simulink model "AVIC_model"  (R2015b)
settings: Solver=ode45  StartTime=0.0  StopTime=simtime  RelTol=1e-3
values from neighbouring files (symbols this model uses):
  A = 1    [simulation.m]
  a1 = 1    [simulation.m]
  a2 = 3    [simulation.m]
  a3 = 3    [simulation.m]
  Amp1 = Ampl/1000000    (= 134.217728)    [simulation.m]
  b1 = 1    [simulation.m]
  B2 = 8    [simulation.m]
  C = 32    [simulation.m]
  c1 = 1    [simulation.m]
  c2 = 1    [simulation.m]
  c3 = 1    [simulation.m]
  finrad = 2*pi/(N)*f0*clk    [simulation.m]
  FSC = 2^27    (= 134217728)    [simulation.m]
  SAT = 127    [simulation.m]
  Ts = 1/clk    (= 1.62760416667e-07)    [simulation.m]
libraries: simulink x298
(part 5 of 5)

== system AVIC_model/2値3次 NSDEM/NSDEM_3rd/Sort16/XSW23 ==
  IP : Inport
  IM : Inport  Port=2
  SP : Inport  Port=3
  SM : Inport  Port=4
  Relational Operator : RelationalOperator  Operator=<  OutDataTypeStr=boolean
  Switch{,1..3} (4 alike) : Switch  Criteria=u2 > Threshold
  OA : Outport
  OB : Outport  Port=2
  QA : Outport  Port=3
  QB : Outport  Port=4
  wires:
  IP/1 -> Relational Operator/1, Switch/1, Switch1/3
  IM/1 -> Relational Operator/2, Switch1/1, Switch/3
  Relational Operator/1 -> Switch/2, Switch1/2, Switch2/2, Switch3/2
  Switch/1 -> OA/1
  Switch1/1 -> OB/1
  SP/1 -> Switch3/3, Switch2/1
  SM/1 -> Switch3/1, Switch2/3
  Switch2/1 -> QA/1
  Switch3/1 -> QB/1

== system AVIC_model/2値3次 NSDEM/NSDEM_3rd/Sort16/XSW24 ==
  IP : Inport
  IM : Inport  Port=2
  SP : Inport  Port=3
  SM : Inport  Port=4
  Relational Operator : RelationalOperator  Operator=<  OutDataTypeStr=boolean
  Switch{,1..3} (4 alike) : Switch  Criteria=u2 > Threshold
  OA : Outport
  OB : Outport  Port=2
  QA : Outport  Port=3
  QB : Outport  Port=4
  wires:
  Switch3/1 -> QB/1
  Switch2/1 -> QA/1
  SM/1 -> Switch2/3, Switch3/1
  SP/1 -> Switch2/1, Switch3/3
  Switch1/1 -> OB/1
  Switch/1 -> OA/1
  Relational Operator/1 -> Switch3/2, Switch2/2, Switch1/2, Switch/2
  IM/1 -> Switch/3, Switch1/1, Relational Operator/2
  IP/1 -> Switch1/3, Switch/1, Relational Operator/1

== system AVIC_model/2値3次 NSDEM/NSDEM_3rd/Sort16/XSW25 ==
  IM : Inport
  IP : Inport  Port=2
  SM : Inport  Port=3
  SP : Inport  Port=4
  Relational Operator : RelationalOperator  Operator=<  OutDataTypeStr=boolean
  Switch{,1..3} (4 alike) : Switch  Criteria=u2 > Threshold
  OB : Outport
  OA : Outport  Port=2
  QB : Outport  Port=3
  QA : Outport  Port=4
  wires:
  IP/1 -> Relational Operator/1, Switch/1, Switch1/3
  IM/1 -> Relational Operator/2, Switch1/1, Switch/3
  Relational Operator/1 -> Switch/2, Switch1/2, Switch2/2, Switch3/2
  Switch/1 -> OA/1
  Switch1/1 -> OB/1
  SP/1 -> Switch3/3, Switch2/1
  SM/1 -> Switch3/1, Switch2/3
  Switch2/1 -> QA/1
  Switch3/1 -> QB/1

== system AVIC_model/2値3次 NSDEM/NSDEM_3rd/Sort16/XSW26 ==
  IM : Inport
  IP : Inport  Port=2
  SM : Inport  Port=3
  SP : Inport  Port=4
  Relational Operator : RelationalOperator  Operator=<  OutDataTypeStr=boolean
  Switch{,1..3} (4 alike) : Switch  Criteria=u2 > Threshold
  OB : Outport
  OA : Outport  Port=2
  QB : Outport  Port=3
  QA : Outport  Port=4
  wires:
  IP/1 -> Relational Operator/1, Switch/1, Switch1/3
  IM/1 -> Relational Operator/2, Switch1/1, Switch/3
  Relational Operator/1 -> Switch/2, Switch1/2, Switch2/2, Switch3/2
  Switch/1 -> OA/1
  Switch1/1 -> OB/1
  SP/1 -> Switch3/3, Switch2/1
  SM/1 -> Switch3/1, Switch2/3
  Switch2/1 -> QA/1
  Switch3/1 -> QB/1

== system AVIC_model/2値3次 NSDEM/NSDEM_3rd/Sort16/XSW27 ==
  IM : Inport
  IP : Inport  Port=2
  SM : Inport  Port=3
  SP : Inport  Port=4
  Relational Operator : RelationalOperator  Operator=<  OutDataTypeStr=boolean
  Switch{,1..3} (4 alike) : Switch  Criteria=u2 > Threshold
  OB : Outport
  OA : Outport  Port=2
  QB : Outport  Port=3
  QA : Outport  Port=4
  wires:
  Switch3/1 -> QB/1
  Switch2/1 -> QA/1
  SM/1 -> Switch2/3, Switch3/1
  SP/1 -> Switch2/1, Switch3/3
  Switch1/1 -> OB/1
  Switch/1 -> OA/1
  Relational Operator/1 -> Switch3/2, Switch2/2, Switch1/2, Switch/2
  IM/1 -> Switch/3, Switch1/1, Relational Operator/2
  IP/1 -> Switch1/3, Switch/1, Relational Operator/1

== system AVIC_model/2値3次 NSDEM/NSDEM_3rd/Sort16/XSW28 ==
  IM : Inport
  IP : Inport  Port=2
  SM : Inport  Port=3
  SP : Inport  Port=4
  Relational Operator : RelationalOperator  Operator=<  OutDataTypeStr=boolean
  Switch{,1..3} (4 alike) : Switch  Criteria=u2 > Threshold
  OB : Outport
  OA : Outport  Port=2
  QB : Outport  Port=3
  QA : Outport  Port=4
  wires:
  Switch3/1 -> QB/1
  Switch2/1 -> QA/1
  SM/1 -> Switch2/3, Switch3/1
  SP/1 -> Switch2/1, Switch3/3
  Switch1/1 -> OB/1
  Switch/1 -> OA/1
  Relational Operator/1 -> Switch3/2, Switch2/2, Switch1/2, Switch/2
  IM/1 -> Switch/3, Switch1/1, Relational Operator/2
  IP/1 -> Switch1/3, Switch/1, Relational Operator/1

== system AVIC_model/2値3次 NSDEM/NSDEM_3rd/Sort16/XSW29 ==
  IM : Inport
  IP : Inport  Port=2
  SM : Inport  Port=3
  SP : Inport  Port=4
  Relational Operator : RelationalOperator  Operator=<  OutDataTypeStr=boolean
  Switch{,1..3} (4 alike) : Switch  Criteria=u2 > Threshold
  OB : Outport
  OA : Outport  Port=2
  QB : Outport  Port=3
  QA : Outport  Port=4
  wires:
  Switch3/1 -> QB/1
  Switch2/1 -> QA/1
  SM/1 -> Switch2/3, Switch3/1
  SP/1 -> Switch2/1, Switch3/3
  Switch1/1 -> OB/1
  Switch/1 -> OA/1
  Relational Operator/1 -> Switch3/2, Switch2/2, Switch1/2, Switch/2
  IM/1 -> Switch/3, Switch1/1, Relational Operator/2
  IP/1 -> Switch1/3, Switch/1, Relational Operator/1

== system AVIC_model/2値3次 NSDEM/NSDEM_3rd/Sort16/XSW3 ==
  IM : Inport
  IP : Inport  Port=2
  SM : Inport  Port=3
  SP : Inport  Port=4
  Relational Operator : RelationalOperator  Operator=<  OutDataTypeStr=boolean
  Switch{,1..3} (4 alike) : Switch  Criteria=u2 > Threshold
  OB : Outport
  OA : Outport  Port=2
  QB : Outport  Port=3
  QA : Outport  Port=4
  wires:
  Switch3/1 -> QB/1
  Switch2/1 -> QA/1
  SM/1 -> Switch2/3, Switch3/1
  SP/1 -> Switch2/1, Switch3/3
  Switch1/1 -> OB/1
  Switch/1 -> OA/1
  Relational Operator/1 -> Switch3/2, Switch2/2, Switch1/2, Switch/2
  IM/1 -> Switch/3, Switch1/1, Relational Operator/2
  IP/1 -> Switch1/3, Switch/1, Relational Operator/1

== system AVIC_model/2値3次 NSDEM/NSDEM_3rd/Sort16/XSW30 ==
  IM : Inport
  IP : Inport  Port=2
  SM : Inport  Port=3
  SP : Inport  Port=4
  Relational Operator : RelationalOperator  Operator=<  OutDataTypeStr=boolean
  Switch{,1..3} (4 alike) : Switch  Criteria=u2 > Threshold
  OB : Outport
  OA : Outport  Port=2
  QB : Outport  Port=3
  QA : Outport  Port=4
  wires:
  Switch3/1 -> QB/1
  Switch2/1 -> QA/1
  SM/1 -> Switch2/3, Switch3/1
  SP/1 -> Switch2/1, Switch3/3
  Switch1/1 -> OB/1
  Switch/1 -> OA/1
  Relational Operator/1 -> Switch3/2, Switch2/2, Switch1/2, Switch/2
  IM/1 -> Switch/3, Switch1/1, Relational Operator/2
  IP/1 -> Switch1/3, Switch/1, Relational Operator/1

== system AVIC_model/2値3次 NSDEM/NSDEM_3rd/Sort16/XSW31 ==
  IM : Inport
  IP : Inport  Port=2
  SM : Inport  Port=3
  SP : Inport  Port=4
  Relational Operator : RelationalOperator  Operator=<  OutDataTypeStr=boolean
  Switch{,1..3} (4 alike) : Switch  Criteria=u2 > Threshold
  OB : Outport
  OA : Outport  Port=2
  QB : Outport  Port=3
  QA : Outport  Port=4
  wires:
  Switch3/1 -> QB/1
  Switch2/1 -> QA/1
  SM/1 -> Switch2/3, Switch3/1
  SP/1 -> Switch2/1, Switch3/3
  Switch1/1 -> OB/1
  Switch/1 -> OA/1
  Relational Operator/1 -> Switch3/2, Switch2/2, Switch1/2, Switch/2
  IM/1 -> Switch/3, Switch1/1, Relational Operator/2
  IP/1 -> Switch1/3, Switch/1, Relational Operator/1

== system AVIC_model/2値3次 NSDEM/NSDEM_3rd/Sort16/XSW32 ==
  IM : Inport
  IP : Inport  Port=2
  SM : Inport  Port=3
  SP : Inport  Port=4
  Relational Operator : RelationalOperator  Operator=<  OutDataTypeStr=boolean
  Switch{,1..3} (4 alike) : Switch  Criteria=u2 > Threshold
  OB : Outport
  OA : Outport  Port=2
  QB : Outport  Port=3
  QA : Outport  Port=4
  wires:
  Switch3/1 -> QB/1
  Switch2/1 -> QA/1
  SM/1 -> Switch2/3, Switch3/1
  SP/1 -> Switch2/1, Switch3/3
  Switch1/1 -> OB/1
  Switch/1 -> OA/1
  Relational Operator/1 -> Switch3/2, Switch2/2, Switch1/2, Switch/2
  IM/1 -> Switch/3, Switch1/1, Relational Operator/2
  IP/1 -> Switch1/3, Switch/1, Relational Operator/1

== system AVIC_model/2値3次 NSDEM/NSDEM_3rd/Sort16/XSW33 ==
  IM : Inport
  IP : Inport  Port=2
  SM : Inport  Port=3
  SP : Inport  Port=4
  Relational Operator : RelationalOperator  Operator=<  OutDataTypeStr=boolean
  Switch{,1..3} (4 alike) : Switch  Criteria=u2 > Threshold
  OB : Outport
  OA : Outport  Port=2
  QB : Outport  Port=3
  QA : Outport  Port=4
  wires:
  Switch3/1 -> QB/1
  Switch2/1 -> QA/1
  SM/1 -> Switch2/3, Switch3/1
  SP/1 -> Switch2/1, Switch3/3
  Switch1/1 -> OB/1
  Switch/1 -> OA/1
  Relational Operator/1 -> Switch3/2, Switch2/2, Switch1/2, Switch/2
  IM/1 -> Switch/3, Switch1/1, Relational Operator/2
  IP/1 -> Switch1/3, Switch/1, Relational Operator/1

== system AVIC_model/2値3次 NSDEM/NSDEM_3rd/Sort16/XSW34 ==
  IM : Inport
  IP : Inport  Port=2
  SM : Inport  Port=3
  SP : Inport  Port=4
  Relational Operator : RelationalOperator  Operator=<  OutDataTypeStr=boolean
  Switch{,1..3} (4 alike) : Switch  Criteria=u2 > Threshold
  OB : Outport
  OA : Outport  Port=2
  QB : Outport  Port=3
  QA : Outport  Port=4
  wires:
  Switch3/1 -> QB/1
  Switch2/1 -> QA/1
  SM/1 -> Switch2/3, Switch3/1
  SP/1 -> Switch2/1, Switch3/3
  Switch1/1 -> OB/1
  Switch/1 -> OA/1
  Relational Operator/1 -> Switch3/2, Switch2/2, Switch1/2, Switch/2
  IM/1 -> Switch/3, Switch1/1, Relational Operator/2
  IP/1 -> Switch1/3, Switch/1, Relational Operator/1

== system AVIC_model/2値3次 NSDEM/NSDEM_3rd/Sort16/XSW35 ==
  IM : Inport
  IP : Inport  Port=2
  SM : Inport  Port=3
  SP : Inport  Port=4
  Relational Operator : RelationalOperator  Operator=<  OutDataTypeStr=boolean
  Switch{,1..3} (4 alike) : Switch  Criteria=u2 > Threshold
  OB : Outport
  OA : Outport  Port=2
  QB : Outport  Port=3
  QA : Outport  Port=4
  wires:
  Switch3/1 -> QB/1
  Switch2/1 -> QA/1
  SM/1 -> Switch2/3, Switch3/1
  SP/1 -> Switch2/1, Switch3/3
  Switch1/1 -> OB/1
  Switch/1 -> OA/1
  Relational Operator/1 -> Switch3/2, Switch2/2, Switch1/2, Switch/2
  IM/1 -> Switch/3, Switch1/1, Relational Operator/2
  IP/1 -> Switch1/3, Switch/1, Relational Operator/1

== system AVIC_model/2値3次 NSDEM/NSDEM_3rd/Sort16/XSW36 ==
  IP : Inport
  IM : Inport  Port=2
  SP : Inport  Port=3
  SM : Inport  Port=4
  Relational Operator : RelationalOperator  Operator=<  OutDataTypeStr=boolean
  Switch{,1..3} (4 alike) : Switch  Criteria=u2 > Threshold
  OA : Outport
  OB : Outport  Port=2
  QA : Outport  Port=3
  QB : Outport  Port=4
  wires:
  IP/1 -> Relational Operator/1, Switch/1, Switch1/3
  IM/1 -> Relational Operator/2, Switch1/1, Switch/3
  Relational Operator/1 -> Switch/2, Switch1/2, Switch2/2, Switch3/2
  Switch/1 -> OA/1
  Switch1/1 -> OB/1
  SP/1 -> Switch3/3, Switch2/1
  SM/1 -> Switch3/1, Switch2/3
  Switch2/1 -> QA/1
  Switch3/1 -> QB/1

== system AVIC_model/2値3次 NSDEM/NSDEM_3rd/Sort16/XSW37 ==
  IM : Inport
  IP : Inport  Port=2
  SM : Inport  Port=3
  SP : Inport  Port=4
  Relational Operator : RelationalOperator  Operator=<  OutDataTypeStr=boolean
  Switch{,1..3} (4 alike) : Switch  Criteria=u2 > Threshold
  OB : Outport
  OA : Outport  Port=2
  QB : Outport  Port=3
  QA : Outport  Port=4
  wires:
  Switch3/1 -> QB/1
  Switch2/1 -> QA/1
  SM/1 -> Switch2/3, Switch3/1
  SP/1 -> Switch2/1, Switch3/3
  Switch1/1 -> OB/1
  Switch/1 -> OA/1
  Relational Operator/1 -> Switch3/2, Switch2/2, Switch1/2, Switch/2
  IM/1 -> Switch/3, Switch1/1, Relational Operator/2
  IP/1 -> Switch1/3, Switch/1, Relational Operator/1

== system AVIC_model/2値3次 NSDEM/NSDEM_3rd/Sort16/XSW38 ==
  IM : Inport
  IP : Inport  Port=2
  SM : Inport  Port=3
  SP : Inport  Port=4
  Relational Operator : RelationalOperator  Operator=<  OutDataTypeStr=boolean
  Switch{,1..3} (4 alike) : Switch  Criteria=u2 > Threshold
  OB : Outport
  OA : Outport  Port=2
  QB : Outport  Port=3
  QA : Outport  Port=4
  wires:
  Switch3/1 -> QB/1
  Switch2/1 -> QA/1
  SM/1 -> Switch2/3, Switch3/1
  SP/1 -> Switch2/1, Switch3/3
  Switch1/1 -> OB/1
  Switch/1 -> OA/1
  Relational Operator/1 -> Switch3/2, Switch2/2, Switch1/2, Switch/2
  IM/1 -> Switch/3, Switch1/1, Relational Operator/2
  IP/1 -> Switch1/3, Switch/1, Relational Operator/1

== system AVIC_model/2値3次 NSDEM/NSDEM_3rd/Sort16/XSW39 ==
  IP : Inport
  IM : Inport  Port=2
  SP : Inport  Port=3
  SM : Inport  Port=4
  Relational Operator : RelationalOperator  Operator=<  OutDataTypeStr=boolean
  Switch{,1..3} (4 alike) : Switch  Criteria=u2 > Threshold
  OA : Outport
  OB : Outport  Port=2
  QA : Outport  Port=3
  QB : Outport  Port=4
  wires:
  Switch3/1 -> QB/1
  Switch2/1 -> QA/1
  SM/1 -> Switch2/3, Switch3/1
  SP/1 -> Switch2/1, Switch3/3
  Switch1/1 -> OB/1
  Switch/1 -> OA/1
  Relational Operator/1 -> Switch3/2, Switch2/2, Switch1/2, Switch/2
  IM/1 -> Switch/3, Switch1/1, Relational Operator/2
  IP/1 -> Switch1/3, Switch/1, Relational Operator/1

== system AVIC_model/2値3次 NSDEM/NSDEM_3rd/Sort16/XSW4 ==
  IP : Inport
  IM : Inport  Port=2
  SP : Inport  Port=3
  SM : Inport  Port=4
  Relational Operator : RelationalOperator  Operator=<  OutDataTypeStr=boolean
  Switch{,1..3} (4 alike) : Switch  Criteria=u2 > Threshold
  OA : Outport
  OB : Outport  Port=2
  QA : Outport  Port=3
  QB : Outport  Port=4
  wires:
  IP/1 -> Relational Operator/1, Switch/1, Switch1/3
  IM/1 -> Relational Operator/2, Switch1/1, Switch/3
  Relational Operator/1 -> Switch/2, Switch1/2, Switch2/2, Switch3/2
  Switch/1 -> OA/1
  Switch1/1 -> OB/1
  SP/1 -> Switch3/3, Switch2/1
  SM/1 -> Switch3/1, Switch2/3
  Switch2/1 -> QA/1
  Switch3/1 -> QB/1

== system AVIC_model/2値3次 NSDEM/NSDEM_3rd/Sort16/XSW40 ==
  IP : Inport
  IM : Inport  Port=2
  SP : Inport  Port=3
  SM : Inport  Port=4
  Relational Operator : RelationalOperator  Operator=<  OutDataTypeStr=boolean
  Switch{,1..3} (4 alike) : Switch  Criteria=u2 > Threshold
  OA : Outport
  OB : Outport  Port=2
  QA : Outport  Port=3
  QB : Outport  Port=4
  wires:
  Switch3/1 -> QB/1
  Switch2/1 -> QA/1
  SM/1 -> Switch2/3, Switch3/1
  SP/1 -> Switch2/1, Switch3/3
  Switch1/1 -> OB/1
  Switch/1 -> OA/1
  Relational Operator/1 -> Switch3/2, Switch2/2, Switch1/2, Switch/2
  IM/1 -> Switch/3, Switch1/1, Relational Operator/2
  IP/1 -> Switch1/3, Switch/1, Relational Operator/1

== system AVIC_model/2値3次 NSDEM/NSDEM_3rd/Sort16/XSW41 ==
  IM : Inport
  IP : Inport  Port=2
  SM : Inport  Port=3
  SP : Inport  Port=4
  Relational Operator : RelationalOperator  Operator=<  OutDataTypeStr=boolean
  Switch{,1..3} (4 alike) : Switch  Criteria=u2 > Threshold
  OB : Outport
  OA : Outport  Port=2
  QB : Outport  Port=3
  QA : Outport  Port=4
  wires:
  Switch3/1 -> QB/1
  Switch2/1 -> QA/1
  SM/1 -> Switch2/3, Switch3/1
  SP/1 -> Switch2/1, Switch3/3
  Switch1/1 -> OB/1
  Switch/1 -> OA/1
  Relational Operator/1 -> Switch3/2, Switch2/2, Switch1/2, Switch/2
  IM/1 -> Switch/3, Switch1/1, Relational Operator/2
  IP/1 -> Switch1/3, Switch/1, Relational Operator/1

== system AVIC_model/2値3次 NSDEM/NSDEM_3rd/Sort16/XSW42 ==
  IP : Inport
  IM : Inport  Port=2
  SP : Inport  Port=3
  SM : Inport  Port=4
  Relational Operator : RelationalOperator  Operator=<  OutDataTypeStr=boolean
  Switch{,1..3} (4 alike) : Switch  Criteria=u2 > Threshold
  OA : Outport
  OB : Outport  Port=2
  QA : Outport  Port=3
  QB : Outport  Port=4
  wires:
  IP/1 -> Relational Operator/1, Switch/1, Switch1/3
  IM/1 -> Relational Operator/2, Switch1/1, Switch/3
  Relational Operator/1 -> Switch/2, Switch1/2, Switch2/2, Switch3/2
  Switch/1 -> OA/1
  Switch1/1 -> OB/1
  SP/1 -> Switch3/3, Switch2/1
  SM/1 -> Switch3/1, Switch2/3
  Switch2/1 -> QA/1
  Switch3/1 -> QB/1

== system AVIC_model/2値3次 NSDEM/NSDEM_3rd/Sort16/XSW43 ==
  IP : Inport
  IM : Inport  Port=2
  SP : Inport  Port=3
  SM : Inport  Port=4
  Relational Operator : RelationalOperator  Operator=<  OutDataTypeStr=boolean
  Switch{,1..3} (4 alike) : Switch  Criteria=u2 > Threshold
  OA : Outport
  OB : Outport  Port=2
  QA : Outport  Port=3
  QB : Outport  Port=4
  wires:
  Switch3/1 -> QB/1
  Switch2/1 -> QA/1
  SM/1 -> Switch2/3, Switch3/1
  SP/1 -> Switch2/1, Switch3/3
  Switch1/1 -> OB/1
  Switch/1 -> OA/1
  Relational Operator/1 -> Switch3/2, Switch2/2, Switch1/2, Switch/2
  IM/1 -> Switch/3, Switch1/1, Relational Operator/2
  IP/1 -> Switch1/3, Switch/1, Relational Operator/1

== system AVIC_model/2値3次 NSDEM/NSDEM_3rd/Sort16/XSW44 ==
  IM : Inport
  IP : Inport  Port=2
  SM : Inport  Port=3
  SP : Inport  Port=4
  Relational Operator : RelationalOperator  Operator=<  OutDataTypeStr=boolean
  Switch{,1..3} (4 alike) : Switch  Criteria=u2 > Threshold
  OB : Outport
  OA : Outport  Port=2
  QB : Outport  Port=3
  QA : Outport  Port=4
  wires:
  Switch3/1 -> QB/1
  Switch2/1 -> QA/1
  SM/1 -> Switch2/3, Switch3/1
  SP/1 -> Switch2/1, Switch3/3
  Switch1/1 -> OB/1
  Switch/1 -> OA/1
  Relational Operator/1 -> Switch3/2, Switch2/2, Switch1/2, Switch/2
  IM/1 -> Switch/3, Switch1/1, Relational Operator/2
  IP/1 -> Switch1/3, Switch/1, Relational Operator/1

== system AVIC_model/2値3次 NSDEM/NSDEM_3rd/Sort16/XSW45 ==
  IM : Inport
  IP : Inport  Port=2
  SM : Inport  Port=3
  SP : Inport  Port=4
  Relational Operator : RelationalOperator  Operator=<  OutDataTypeStr=boolean
  Switch{,1..3} (4 alike) : Switch  Criteria=u2 > Threshold
  OB : Outport
  OA : Outport  Port=2
  QB : Outport  Port=3
  QA : Outport  Port=4
  wires:
  IP/1 -> Relational Operator/1, Switch/1, Switch1/3
  IM/1 -> Relational Operator/2, Switch1/1, Switch/3
  Relational Operator/1 -> Switch/2, Switch1/2, Switch2/2, Switch3/2
  Switch/1 -> OA/1
  Switch1/1 -> OB/1
  SP/1 -> Switch3/3, Switch2/1
  SM/1 -> Switch3/1, Switch2/3
  Switch2/1 -> QA/1
  Switch3/1 -> QB/1

== system AVIC_model/2値3次 NSDEM/NSDEM_3rd/Sort16/XSW46 ==
  IP : Inport
  IM : Inport  Port=2
  SP : Inport  Port=3
  SM : Inport  Port=4
  Relational Operator : RelationalOperator  Operator=<  OutDataTypeStr=boolean
  Switch{,1..3} (4 alike) : Switch  Criteria=u2 > Threshold
  OA : Outport
  OB : Outport  Port=2
  QA : Outport  Port=3
  QB : Outport  Port=4
  wires:
  Switch3/1 -> QB/1
  Switch2/1 -> QA/1
  SM/1 -> Switch2/3, Switch3/1
  SP/1 -> Switch2/1, Switch3/3
  Switch1/1 -> OB/1
  Switch/1 -> OA/1
  Relational Operator/1 -> Switch3/2, Switch2/2, Switch1/2, Switch/2
  IM/1 -> Switch/3, Switch1/1, Relational Operator/2
  IP/1 -> Switch1/3, Switch/1, Relational Operator/1

== system AVIC_model/2値3次 NSDEM/NSDEM_3rd/Sort16/XSW47 ==
  IP : Inport
  IM : Inport  Port=2
  SP : Inport  Port=3
  SM : Inport  Port=4
  Relational Operator : RelationalOperator  Operator=<  OutDataTypeStr=boolean
  Switch{,1..3} (4 alike) : Switch  Criteria=u2 > Threshold
  OA : Outport
  OB : Outport  Port=2
  QA : Outport  Port=3
  QB : Outport  Port=4
  wires:
  IP/1 -> Relational Operator/1, Switch/1, Switch1/3
  IM/1 -> Relational Operator/2, Switch1/1, Switch/3
  Relational Operator/1 -> Switch/2, Switch1/2, Switch2/2, Switch3/2
  Switch/1 -> OA/1
  Switch1/1 -> OB/1
  SP/1 -> Switch3/3, Switch2/1
  SM/1 -> Switch3/1, Switch2/3
  Switch2/1 -> QA/1
  Switch3/1 -> QB/1

== system AVIC_model/2値3次 NSDEM/NSDEM_3rd/Sort16/XSW48 ==
  IP : Inport
  IM : Inport  Port=2
  SP : Inport  Port=3
  SM : Inport  Port=4
  Relational Operator : RelationalOperator  Operator=<  OutDataTypeStr=boolean
  Switch{,1..3} (4 alike) : Switch  Criteria=u2 > Threshold
  OA : Outport
  OB : Outport  Port=2
  QA : Outport  Port=3
  QB : Outport  Port=4
  wires:
  Switch3/1 -> QB/1
  Switch2/1 -> QA/1
  SM/1 -> Switch2/3, Switch3/1
  SP/1 -> Switch2/1, Switch3/3
  Switch1/1 -> OB/1
  Switch/1 -> OA/1
  Relational Operator/1 -> Switch3/2, Switch2/2, Switch1/2, Switch/2
  IM/1 -> Switch/3, Switch1/1, Relational Operator/2
  IP/1 -> Switch1/3, Switch/1, Relational Operator/1

== system AVIC_model/2値3次 NSDEM/NSDEM_3rd/Sort16/XSW49 ==
  IP : Inport
  IM : Inport  Port=2
  SP : Inport  Port=3
  SM : Inport  Port=4
  Relational Operator : RelationalOperator  Operator=<  OutDataTypeStr=boolean
  Switch{,1..3} (4 alike) : Switch  Criteria=u2 > Threshold
  OA : Outport
  OB : Outport  Port=2
  QA : Outport  Port=3
  QB : Outport  Port=4
  wires:
  Switch3/1 -> QB/1
  Switch2/1 -> QA/1
  SM/1 -> Switch2/3, Switch3/1
  SP/1 -> Switch2/1, Switch3/3
  Switch1/1 -> OB/1
  Switch/1 -> OA/1
  Relational Operator/1 -> Switch3/2, Switch2/2, Switch1/2, Switch/2
  IM/1 -> Switch/3, Switch1/1, Relational Operator/2
  IP/1 -> Switch1/3, Switch/1, Relational Operator/1

== system AVIC_model/2値3次 NSDEM/NSDEM_3rd/Sort16/XSW5 ==
  IP : Inport
  IM : Inport  Port=2
  SP : Inport  Port=3
  SM : Inport  Port=4
  Relational Operator : RelationalOperator  Operator=<  OutDataTypeStr=boolean
  Switch{,1..3} (4 alike) : Switch  Criteria=u2 > Threshold
  OA : Outport
  OB : Outport  Port=2
  QA : Outport  Port=3
  QB : Outport  Port=4
  wires:
  Switch3/1 -> QB/1
  Switch2/1 -> QA/1
  SM/1 -> Switch2/3, Switch3/1
  SP/1 -> Switch2/1, Switch3/3
  Switch1/1 -> OB/1
  Switch/1 -> OA/1
  Relational Operator/1 -> Switch3/2, Switch2/2, Switch1/2, Switch/2
  IM/1 -> Switch/3, Switch1/1, Relational Operator/2
  IP/1 -> Switch1/3, Switch/1, Relational Operator/1

== system AVIC_model/2値3次 NSDEM/NSDEM_3rd/Sort16/XSW50 ==
  IP : Inport
  IM : Inport  Port=2
  SP : Inport  Port=3
  SM : Inport  Port=4
  Relational Operator : RelationalOperator  Operator=<  OutDataTypeStr=boolean
  Switch{,1..3} (4 alike) : Switch  Criteria=u2 > Threshold
  OA : Outport
  OB : Outport  Port=2
  QA : Outport  Port=3
  QB : Outport  Port=4
  wires:
  Switch3/1 -> QB/1
  Switch2/1 -> QA/1
  SM/1 -> Switch2/3, Switch3/1
  SP/1 -> Switch2/1, Switch3/3
  Switch1/1 -> OB/1
  Switch/1 -> OA/1
  Relational Operator/1 -> Switch3/2, Switch2/2, Switch1/2, Switch/2
  IM/1 -> Switch/3, Switch1/1, Relational Operator/2
  IP/1 -> Switch1/3, Switch/1, Relational Operator/1

== system AVIC_model/2値3次 NSDEM/NSDEM_3rd/Sort16/XSW51 ==
  IP : Inport
  IM : Inport  Port=2
  SP : Inport  Port=3
  SM : Inport  Port=4
  Relational Operator : RelationalOperator  Operator=<  OutDataTypeStr=boolean
  Switch{,1..3} (4 alike) : Switch  Criteria=u2 > Threshold
  OA : Outport
  OB : Outport  Port=2
  QA : Outport  Port=3
  QB : Outport  Port=4
  wires:
  Switch3/1 -> QB/1
  Switch2/1 -> QA/1
  SM/1 -> Switch2/3, Switch3/1
  SP/1 -> Switch2/1, Switch3/3
  Switch1/1 -> OB/1
  Switch/1 -> OA/1
  Relational Operator/1 -> Switch3/2, Switch2/2, Switch1/2, Switch/2
  IM/1 -> Switch/3, Switch1/1, Relational Operator/2
  IP/1 -> Switch1/3, Switch/1, Relational Operator/1

== system AVIC_model/2値3次 NSDEM/NSDEM_3rd/Sort16/XSW52 ==
  IP : Inport
  IM : Inport  Port=2
  SP : Inport  Port=3
  SM : Inport  Port=4
  Relational Operator : RelationalOperator  Operator=<  OutDataTypeStr=boolean
  Switch{,1..3} (4 alike) : Switch  Criteria=u2 > Threshold
  OA : Outport
  OB : Outport  Port=2
  QA : Outport  Port=3
  QB : Outport  Port=4
  wires:
  Switch3/1 -> QB/1
  Switch2/1 -> QA/1
  SM/1 -> Switch2/3, Switch3/1
  SP/1 -> Switch2/1, Switch3/3
  Switch1/1 -> OB/1
  Switch/1 -> OA/1
  Relational Operator/1 -> Switch3/2, Switch2/2, Switch1/2, Switch/2
  IM/1 -> Switch/3, Switch1/1, Relational Operator/2
  IP/1 -> Switch1/3, Switch/1, Relational Operator/1

== system AVIC_model/2値3次 NSDEM/NSDEM_3rd/Sort16/XSW53 ==
  IP : Inport
  IM : Inport  Port=2
  SP : Inport  Port=3
  SM : Inport  Port=4
  Relational Operator : RelationalOperator  Operator=<  OutDataTypeStr=boolean
  Switch{,1..3} (4 alike) : Switch  Criteria=u2 > Threshold
  OA : Outport
  OB : Outport  Port=2
  QA : Outport  Port=3
  QB : Outport  Port=4
  wires:
  Switch3/1 -> QB/1
  Switch2/1 -> QA/1
  SM/1 -> Switch2/3, Switch3/1
  SP/1 -> Switch2/1, Switch3/3
  Switch1/1 -> OB/1
  Switch/1 -> OA/1
  Relational Operator/1 -> Switch3/2, Switch2/2, Switch1/2, Switch/2
  IM/1 -> Switch/3, Switch1/1, Relational Operator/2
  IP/1 -> Switch1/3, Switch/1, Relational Operator/1

== system AVIC_model/2値3次 NSDEM/NSDEM_3rd/Sort16/XSW54 ==
  IP : Inport
  IM : Inport  Port=2
  SP : Inport  Port=3
  SM : Inport  Port=4
  Relational Operator : RelationalOperator  Operator=<  OutDataTypeStr=boolean
  Switch{,1..3} (4 alike) : Switch  Criteria=u2 > Threshold
  OA : Outport
  OB : Outport  Port=2
  QA : Outport  Port=3
  QB : Outport  Port=4
  wires:
  Switch3/1 -> QB/1
  Switch2/1 -> QA/1
  SM/1 -> Switch2/3, Switch3/1
  SP/1 -> Switch2/1, Switch3/3
  Switch1/1 -> OB/1
  Switch/1 -> OA/1
  Relational Operator/1 -> Switch3/2, Switch2/2, Switch1/2, Switch/2
  IM/1 -> Switch/3, Switch1/1, Relational Operator/2
  IP/1 -> Switch1/3, Switch/1, Relational Operator/1

== system AVIC_model/2値3次 NSDEM/NSDEM_3rd/Sort16/XSW55 ==
  IP : Inport
  IM : Inport  Port=2
  SP : Inport  Port=3
  SM : Inport  Port=4
  Relational Operator : RelationalOperator  Operator=<  OutDataTypeStr=boolean
  Switch{,1..3} (4 alike) : Switch  Criteria=u2 > Threshold
  OA : Outport
  OB : Outport  Port=2
  QA : Outport  Port=3
  QB : Outport  Port=4
  wires:
  IP/1 -> Relational Operator/1, Switch/1, Switch1/3
  IM/1 -> Relational Operator/2, Switch1/1, Switch/3
  Relational Operator/1 -> Switch/2, Switch1/2, Switch2/2, Switch3/2
  Switch/1 -> OA/1
  Switch1/1 -> OB/1
  SP/1 -> Switch3/3, Switch2/1
  SM/1 -> Switch3/1, Switch2/3
  Switch2/1 -> QA/1
  Switch3/1 -> QB/1

== system AVIC_model/2値3次 NSDEM/NSDEM_3rd/Sort16/XSW56 ==
  IP : Inport
  IM : Inport  Port=2
  SP : Inport  Port=3
  SM : Inport  Port=4
  Relational Operator : RelationalOperator  Operator=<  OutDataTypeStr=boolean
  Switch{,1..3} (4 alike) : Switch  Criteria=u2 > Threshold
  OA : Outport
  OB : Outport  Port=2
  QA : Outport  Port=3
  QB : Outport  Port=4
  wires:
  Switch3/1 -> QB/1
  Switch2/1 -> QA/1
  SM/1 -> Switch2/3, Switch3/1
  SP/1 -> Switch2/1, Switch3/3
  Switch1/1 -> OB/1
  Switch/1 -> OA/1
  Relational Operator/1 -> Switch3/2, Switch2/2, Switch1/2, Switch/2
  IM/1 -> Switch/3, Switch1/1, Relational Operator/2
  IP/1 -> Switch1/3, Switch/1, Relational Operator/1

== system AVIC_model/2値3次 NSDEM/NSDEM_3rd/Sort16/XSW57 ==
  IP : Inport
  IM : Inport  Port=2
  SP : Inport  Port=3
  SM : Inport  Port=4
  Relational Operator : RelationalOperator  Operator=<  OutDataTypeStr=boolean
  Switch{,1..3} (4 alike) : Switch  Criteria=u2 > Threshold
  OA : Outport
  OB : Outport  Port=2
  QA : Outport  Port=3
  QB : Outport  Port=4
  wires:
  IP/1 -> Relational Operator/1, Switch/1, Switch1/3
  IM/1 -> Relational Operator/2, Switch1/1, Switch/3
  Relational Operator/1 -> Switch/2, Switch1/2, Switch2/2, Switch3/2
  Switch/1 -> OA/1
  Switch1/1 -> OB/1
  SP/1 -> Switch3/3, Switch2/1
  SM/1 -> Switch3/1, Switch2/3
  Switch2/1 -> QA/1
  Switch3/1 -> QB/1

== system AVIC_model/2値3次 NSDEM/NSDEM_3rd/Sort16/XSW58 ==
  IP : Inport
  IM : Inport  Port=2
  SP : Inport  Port=3
  SM : Inport  Port=4
  Relational Operator : RelationalOperator  Operator=<  OutDataTypeStr=boolean
  Switch{,1..3} (4 alike) : Switch  Criteria=u2 > Threshold
  OA : Outport
  OB : Outport  Port=2
  QA : Outport  Port=3
  QB : Outport  Port=4
  wires:
  Switch3/1 -> QB/1
  Switch2/1 -> QA/1
  SM/1 -> Switch2/3, Switch3/1
  SP/1 -> Switch2/1, Switch3/3
  Switch1/1 -> OB/1
  Switch/1 -> OA/1
  Relational Operator/1 -> Switch3/2, Switch2/2, Switch1/2, Switch/2
  IM/1 -> Switch/3, Switch1/1, Relational Operator/2
  IP/1 -> Switch1/3, Switch/1, Relational Operator/1

== system AVIC_model/2値3次 NSDEM/NSDEM_3rd/Sort16/XSW59 ==
  IP : Inport
  IM : Inport  Port=2
  SP : Inport  Port=3
  SM : Inport  Port=4
  Relational Operator : RelationalOperator  Operator=<  OutDataTypeStr=boolean
  Switch{,1..3} (4 alike) : Switch  Criteria=u2 > Threshold
  OA : Outport
  OB : Outport  Port=2
  QA : Outport  Port=3
  QB : Outport  Port=4
  wires:
  Switch3/1 -> QB/1
  Switch2/1 -> QA/1
  SM/1 -> Switch2/3, Switch3/1
  SP/1 -> Switch2/1, Switch3/3
  Switch1/1 -> OB/1
  Switch/1 -> OA/1
  Relational Operator/1 -> Switch3/2, Switch2/2, Switch1/2, Switch/2
  IM/1 -> Switch/3, Switch1/1, Relational Operator/2
  IP/1 -> Switch1/3, Switch/1, Relational Operator/1

== system AVIC_model/2値3次 NSDEM/NSDEM_3rd/Sort16/XSW6 ==
  IM : Inport
  IP : Inport  Port=2
  SM : Inport  Port=3
  SP : Inport  Port=4
  Relational Operator : RelationalOperator  Operator=<  OutDataTypeStr=boolean
  Switch{,1..3} (4 alike) : Switch  Criteria=u2 > Threshold
  OB : Outport
  OA : Outport  Port=2
  QB : Outport  Port=3
  QA : Outport  Port=4
  wires:
  Switch3/1 -> QB/1
  Switch2/1 -> QA/1
  SM/1 -> Switch2/3, Switch3/1
  SP/1 -> Switch2/1, Switch3/3
  Switch1/1 -> OB/1
  Switch/1 -> OA/1
  Relational Operator/1 -> Switch3/2, Switch2/2, Switch1/2, Switch/2
  IM/1 -> Switch/3, Switch1/1, Relational Operator/2
  IP/1 -> Switch1/3, Switch/1, Relational Operator/1

== system AVIC_model/2値3次 NSDEM/NSDEM_3rd/Sort16/XSW60 ==
  IP : Inport
  IM : Inport  Port=2
  SP : Inport  Port=3
  SM : Inport  Port=4
  Relational Operator : RelationalOperator  Operator=<  OutDataTypeStr=boolean
  Switch{,1..3} (4 alike) : Switch  Criteria=u2 > Threshold
  OA : Outport
  OB : Outport  Port=2
  QA : Outport  Port=3
  QB : Outport  Port=4
  wires:
  Switch3/1 -> QB/1
  Switch2/1 -> QA/1
  SM/1 -> Switch2/3, Switch3/1
  SP/1 -> Switch2/1, Switch3/3
  Switch1/1 -> OB/1
  Switch/1 -> OA/1
  Relational Operator/1 -> Switch3/2, Switch2/2, Switch1/2, Switch/2
  IM/1 -> Switch/3, Switch1/1, Relational Operator/2
  IP/1 -> Switch1/3, Switch/1, Relational Operator/1

== system AVIC_model/2値3次 NSDEM/NSDEM_3rd/Sort16/XSW61 ==
  IP : Inport
  IM : Inport  Port=2
  SP : Inport  Port=3
  SM : Inport  Port=4
  Relational Operator : RelationalOperator  Operator=<  OutDataTypeStr=boolean
  Switch{,1..3} (4 alike) : Switch  Criteria=u2 > Threshold
  OA : Outport
  OB : Outport  Port=2
  QA : Outport  Port=3
  QB : Outport  Port=4
  wires:
  Switch3/1 -> QB/1
  Switch2/1 -> QA/1
  SM/1 -> Switch2/3, Switch3/1
  SP/1 -> Switch2/1, Switch3/3
  Switch1/1 -> OB/1
  Switch/1 -> OA/1
  Relational Operator/1 -> Switch3/2, Switch2/2, Switch1/2, Switch/2
  IM/1 -> Switch/3, Switch1/1, Relational Operator/2
  IP/1 -> Switch1/3, Switch/1, Relational Operator/1

== system AVIC_model/2値3次 NSDEM/NSDEM_3rd/Sort16/XSW62 ==
  IP : Inport
  IM : Inport  Port=2
  SP : Inport  Port=3
  SM : Inport  Port=4
  Relational Operator : RelationalOperator  Operator=<  OutDataTypeStr=boolean
  Switch{,1..3} (4 alike) : Switch  Criteria=u2 > Threshold
  OA : Outport
  OB : Outport  Port=2
  QA : Outport  Port=3
  QB : Outport  Port=4
  wires:
  Switch3/1 -> QB/1
  Switch2/1 -> QA/1
  SM/1 -> Switch2/3, Switch3/1
  SP/1 -> Switch2/1, Switch3/3
  Switch1/1 -> OB/1
  Switch/1 -> OA/1
  Relational Operator/1 -> Switch3/2, Switch2/2, Switch1/2, Switch/2
  IM/1 -> Switch/3, Switch1/1, Relational Operator/2
  IP/1 -> Switch1/3, Switch/1, Relational Operator/1

== system AVIC_model/2値3次 NSDEM/NSDEM_3rd/Sort16/XSW63 ==
  IP : Inport
  IM : Inport  Port=2
  SP : Inport  Port=3
  SM : Inport  Port=4
  Relational Operator : RelationalOperator  Operator=<  OutDataTypeStr=boolean
  Switch{,1..3} (4 alike) : Switch  Criteria=u2 > Threshold
  OA : Outport
  OB : Outport  Port=2
  QA : Outport  Port=3
  QB : Outport  Port=4
  wires:
  Switch3/1 -> QB/1
  Switch2/1 -> QA/1
  SM/1 -> Switch2/3, Switch3/1
  SP/1 -> Switch2/1, Switch3/3
  Switch1/1 -> OB/1
  Switch/1 -> OA/1
  Relational Operator/1 -> Switch3/2, Switch2/2, Switch1/2, Switch/2
  IM/1 -> Switch/3, Switch1/1, Relational Operator/2
  IP/1 -> Switch1/3, Switch/1, Relational Operator/1

== system AVIC_model/2値3次 NSDEM/NSDEM_3rd/Sort16/XSW64 ==
  IP : Inport
  IM : Inport  Port=2
  SP : Inport  Port=3
  SM : Inport  Port=4
  Relational Operator : RelationalOperator  Operator=<  OutDataTypeStr=boolean
  Switch{,1..3} (4 alike) : Switch  Criteria=u2 > Threshold
  OA : Outport
  OB : Outport  Port=2
  QA : Outport  Port=3
  QB : Outport  Port=4
  wires:
  Switch3/1 -> QB/1
  Switch2/1 -> QA/1
  SM/1 -> Switch2/3, Switch3/1
  SP/1 -> Switch2/1, Switch3/3
  Switch1/1 -> OB/1
  Switch/1 -> OA/1
  Relational Operator/1 -> Switch3/2, Switch2/2, Switch1/2, Switch/2
  IM/1 -> Switch/3, Switch1/1, Relational Operator/2
  IP/1 -> Switch1/3, Switch/1, Relational Operator/1

== system AVIC_model/2値3次 NSDEM/NSDEM_3rd/Sort16/XSW65 ==
  IP : Inport
  IM : Inport  Port=2
  SP : Inport  Port=3
  SM : Inport  Port=4
  Relational Operator : RelationalOperator  Operator=<  OutDataTypeStr=boolean
  Switch{,1..3} (4 alike) : Switch  Criteria=u2 > Threshold
  OA : Outport
  OB : Outport  Port=2
  QA : Outport  Port=3
  QB : Outport  Port=4
  wires:
  IP/1 -> Relational Operator/1, Switch/1, Switch1/3
  IM/1 -> Relational Operator/2, Switch1/1, Switch/3
  Relational Operator/1 -> Switch/2, Switch1/2, Switch2/2, Switch3/2
  Switch/1 -> OA/1
  Switch1/1 -> OB/1
  SP/1 -> Switch3/3, Switch2/1
  SM/1 -> Switch3/1, Switch2/3
  Switch2/1 -> QA/1
  Switch3/1 -> QB/1

== system AVIC_model/2値3次 NSDEM/NSDEM_3rd/Sort16/XSW66 ==
  IP : Inport
  IM : Inport  Port=2
  SP : Inport  Port=3
  SM : Inport  Port=4
  Relational Operator : RelationalOperator  Operator=<  OutDataTypeStr=boolean
  Switch{,1..3} (4 alike) : Switch  Criteria=u2 > Threshold
  OA : Outport
  OB : Outport  Port=2
  QA : Outport  Port=3
  QB : Outport  Port=4
  wires:
  Switch3/1 -> QB/1
  Switch2/1 -> QA/1
  SM/1 -> Switch2/3, Switch3/1
  SP/1 -> Switch2/1, Switch3/3
  Switch1/1 -> OB/1
  Switch/1 -> OA/1
  Relational Operator/1 -> Switch3/2, Switch2/2, Switch1/2, Switch/2
  IM/1 -> Switch/3, Switch1/1, Relational Operator/2
  IP/1 -> Switch1/3, Switch/1, Relational Operator/1

== system AVIC_model/2値3次 NSDEM/NSDEM_3rd/Sort16/XSW67 ==
  IP : Inport
  IM : Inport  Port=2
  SP : Inport  Port=3
  SM : Inport  Port=4
  Relational Operator : RelationalOperator  Operator=<  OutDataTypeStr=boolean
  Switch{,1..3} (4 alike) : Switch  Criteria=u2 > Threshold
  OA : Outport
  OB : Outport  Port=2
  QA : Outport  Port=3
  QB : Outport  Port=4
  wires:
  IP/1 -> Relational Operator/1, Switch/1, Switch1/3
  IM/1 -> Relational Operator/2, Switch1/1, Switch/3
  Relational Operator/1 -> Switch/2, Switch1/2, Switch2/2, Switch3/2
  Switch/1 -> OA/1
  Switch1/1 -> OB/1
  SP/1 -> Switch3/3, Switch2/1
  SM/1 -> Switch3/1, Switch2/3
  Switch2/1 -> QA/1
  Switch3/1 -> QB/1

== system AVIC_model/2値3次 NSDEM/NSDEM_3rd/Sort16/XSW68 ==
  IP : Inport
  IM : Inport  Port=2
  SP : Inport  Port=3
  SM : Inport  Port=4
  Relational Operator : RelationalOperator  Operator=<  OutDataTypeStr=boolean
  Switch{,1..3} (4 alike) : Switch  Criteria=u2 > Threshold
  OA : Outport
  OB : Outport  Port=2
  QA : Outport  Port=3
  QB : Outport  Port=4
  wires:
  Switch3/1 -> QB/1
  Switch2/1 -> QA/1
  SM/1 -> Switch2/3, Switch3/1
  SP/1 -> Switch2/1, Switch3/3
  Switch1/1 -> OB/1
  Switch/1 -> OA/1
  Relational Operator/1 -> Switch3/2, Switch2/2, Switch1/2, Switch/2
  IM/1 -> Switch/3, Switch1/1, Relational Operator/2
  IP/1 -> Switch1/3, Switch/1, Relational Operator/1

== system AVIC_model/2値3次 NSDEM/NSDEM_3rd/Sort16/XSW69 ==
  IP : Inport
  IM : Inport  Port=2
  SP : Inport  Port=3
  SM : Inport  Port=4
  Relational Operator : RelationalOperator  Operator=<  OutDataTypeStr=boolean
  Switch{,1..3} (4 alike) : Switch  Criteria=u2 > Threshold
  OA : Outport
  OB : Outport  Port=2
  QA : Outport  Port=3
  QB : Outport  Port=4
  wires:
  Switch3/1 -> QB/1
  Switch2/1 -> QA/1
  SM/1 -> Switch2/3, Switch3/1
  SP/1 -> Switch2/1, Switch3/3
  Switch1/1 -> OB/1
  Switch/1 -> OA/1
  Relational Operator/1 -> Switch3/2, Switch2/2, Switch1/2, Switch/2
  IM/1 -> Switch/3, Switch1/1, Relational Operator/2
  IP/1 -> Switch1/3, Switch/1, Relational Operator/1

== system AVIC_model/2値3次 NSDEM/NSDEM_3rd/Sort16/XSW7 ==
  IM : Inport
  IP : Inport  Port=2
  SM : Inport  Port=3
  SP : Inport  Port=4
  Relational Operator : RelationalOperator  Operator=<  OutDataTypeStr=boolean
  Switch{,1..3} (4 alike) : Switch  Criteria=u2 > Threshold
  OB : Outport
  OA : Outport  Port=2
  QB : Outport  Port=3
  QA : Outport  Port=4
  wires:
  IP/1 -> Relational Operator/1, Switch/1, Switch1/3
  IM/1 -> Relational Operator/2, Switch1/1, Switch/3
  Relational Operator/1 -> Switch/2, Switch1/2, Switch2/2, Switch3/2
  Switch/1 -> OA/1
  Switch1/1 -> OB/1
  SP/1 -> Switch3/3, Switch2/1
  SM/1 -> Switch3/1, Switch2/3
  Switch2/1 -> QA/1
  Switch3/1 -> QB/1

== system AVIC_model/2値3次 NSDEM/NSDEM_3rd/Sort16/XSW72 ==
  IP : Inport
  IM : Inport  Port=2
  SP : Inport  Port=3
  SM : Inport  Port=4
  Relational Operator : RelationalOperator  Operator=<  OutDataTypeStr=boolean
  Switch{,1..3} (4 alike) : Switch  Criteria=u2 > Threshold
  OA : Outport
  OB : Outport  Port=2
  QA : Outport  Port=3
  QB : Outport  Port=4
  wires:
  Switch3/1 -> QB/1
  Switch2/1 -> QA/1
  SM/1 -> Switch2/3, Switch3/1
  SP/1 -> Switch2/1, Switch3/3
  Switch1/1 -> OB/1
  Switch/1 -> OA/1
  Relational Operator/1 -> Switch3/2, Switch2/2, Switch1/2, Switch/2
  IM/1 -> Switch/3, Switch1/1, Relational Operator/2
  IP/1 -> Switch1/3, Switch/1, Relational Operator/1

== system AVIC_model/2値3次 NSDEM/NSDEM_3rd/Sort16/XSW73 ==
  IP : Inport
  IM : Inport  Port=2
  SP : Inport  Port=3
  SM : Inport  Port=4
  Relational Operator : RelationalOperator  Operator=<  OutDataTypeStr=boolean
  Switch{,1..3} (4 alike) : Switch  Criteria=u2 > Threshold
  OA : Outport
  OB : Outport  Port=2
  QA : Outport  Port=3
  QB : Outport  Port=4
  wires:
  IP/1 -> Relational Operator/1, Switch/1, Switch1/3
  IM/1 -> Relational Operator/2, Switch1/1, Switch/3
  Relational Operator/1 -> Switch/2, Switch1/2, Switch2/2, Switch3/2
  Switch/1 -> OA/1
  Switch1/1 -> OB/1
  SP/1 -> Switch3/3, Switch2/1
  SM/1 -> Switch3/1, Switch2/3
  Switch2/1 -> QA/1
  Switch3/1 -> QB/1

== system AVIC_model/2値3次 NSDEM/NSDEM_3rd/Sort16/XSW74 ==
  IP : Inport
  IM : Inport  Port=2
  SP : Inport  Port=3
  SM : Inport  Port=4
  Relational Operator : RelationalOperator  Operator=<  OutDataTypeStr=boolean
  Switch{,1..3} (4 alike) : Switch  Criteria=u2 > Threshold
  OA : Outport
  OB : Outport  Port=2
  QA : Outport  Port=3
  QB : Outport  Port=4
  wires:
  Switch3/1 -> QB/1
  Switch2/1 -> QA/1
  SM/1 -> Switch2/3, Switch3/1
  SP/1 -> Switch2/1, Switch3/3
  Switch1/1 -> OB/1
  Switch/1 -> OA/1
  Relational Operator/1 -> Switch3/2, Switch2/2, Switch1/2, Switch/2
  IM/1 -> Switch/3, Switch1/1, Relational Operator/2
  IP/1 -> Switch1/3, Switch/1, Relational Operator/1

== system AVIC_model/2値3次 NSDEM/NSDEM_3rd/Sort16/XSW75 ==
  IP : Inport
  IM : Inport  Port=2
  SP : Inport  Port=3
  SM : Inport  Port=4
  Relational Operator : RelationalOperator  Operator=<  OutDataTypeStr=boolean
  Switch{,1..3} (4 alike) : Switch  Criteria=u2 > Threshold
  OA : Outport
  OB : Outport  Port=2
  QA : Outport  Port=3
  QB : Outport  Port=4
  wires:
  IP/1 -> Relational Operator/1, Switch/1, Switch1/3
  IM/1 -> Relational Operator/2, Switch1/1, Switch/3
  Relational Operator/1 -> Switch/2, Switch1/2, Switch2/2, Switch3/2
  Switch/1 -> OA/1
  Switch1/1 -> OB/1
  SP/1 -> Switch3/3, Switch2/1
  SM/1 -> Switch3/1, Switch2/3
  Switch2/1 -> QA/1
  Switch3/1 -> QB/1

== system AVIC_model/2値3次 NSDEM/NSDEM_3rd/Sort16/XSW76 ==
  IP : Inport
  IM : Inport  Port=2
  SP : Inport  Port=3
  SM : Inport  Port=4
  Relational Operator : RelationalOperator  Operator=<  OutDataTypeStr=boolean
  Switch{,1..3} (4 alike) : Switch  Criteria=u2 > Threshold
  OA : Outport
  OB : Outport  Port=2
  QA : Outport  Port=3
  QB : Outport  Port=4
  wires:
  Switch3/1 -> QB/1
  Switch2/1 -> QA/1
  SM/1 -> Switch2/3, Switch3/1
  SP/1 -> Switch2/1, Switch3/3
  Switch1/1 -> OB/1
  Switch/1 -> OA/1
  Relational Operator/1 -> Switch3/2, Switch2/2, Switch1/2, Switch/2
  IM/1 -> Switch/3, Switch1/1, Relational Operator/2
  IP/1 -> Switch1/3, Switch/1, Relational Operator/1

== system AVIC_model/2値3次 NSDEM/NSDEM_3rd/Sort16/XSW77 ==
  IP : Inport
  IM : Inport  Port=2
  SP : Inport  Port=3
  SM : Inport  Port=4
  Relational Operator : RelationalOperator  Operator=<  OutDataTypeStr=boolean
  Switch{,1..3} (4 alike) : Switch  Criteria=u2 > Threshold
  OA : Outport
  OB : Outport  Port=2
  QA : Outport  Port=3
  QB : Outport  Port=4
  wires:
  IP/1 -> Relational Operator/1, Switch/1, Switch1/3
  IM/1 -> Relational Operator/2, Switch1/1, Switch/3
  Relational Operator/1 -> Switch/2, Switch1/2, Switch2/2, Switch3/2
  Switch/1 -> OA/1
  Switch1/1 -> OB/1
  SP/1 -> Switch3/3, Switch2/1
  SM/1 -> Switch3/1, Switch2/3
  Switch2/1 -> QA/1
  Switch3/1 -> QB/1

== system AVIC_model/2値3次 NSDEM/NSDEM_3rd/Sort16/XSW78 ==
  IP : Inport
  IM : Inport  Port=2
  SP : Inport  Port=3
  SM : Inport  Port=4
  Relational Operator : RelationalOperator  Operator=<  OutDataTypeStr=boolean
  Switch{,1..3} (4 alike) : Switch  Criteria=u2 > Threshold
  OA : Outport
  OB : Outport  Port=2
  QA : Outport  Port=3
  QB : Outport  Port=4
  wires:
  Switch3/1 -> QB/1
  Switch2/1 -> QA/1
  SM/1 -> Switch2/3, Switch3/1
  SP/1 -> Switch2/1, Switch3/3
  Switch1/1 -> OB/1
  Switch/1 -> OA/1
  Relational Operator/1 -> Switch3/2, Switch2/2, Switch1/2, Switch/2
  IM/1 -> Switch/3, Switch1/1, Relational Operator/2
  IP/1 -> Switch1/3, Switch/1, Relational Operator/1

== system AVIC_model/2値3次 NSDEM/NSDEM_3rd/Sort16/XSW79 ==
  IP : Inport
  IM : Inport  Port=2
  SP : Inport  Port=3
  SM : Inport  Port=4
  Relational Operator : RelationalOperator  Operator=<  OutDataTypeStr=boolean
  Switch{,1..3} (4 alike) : Switch  Criteria=u2 > Threshold
  OA : Outport
  OB : Outport  Port=2
  QA : Outport  Port=3
  QB : Outport  Port=4
  wires:
  IP/1 -> Relational Operator/1, Switch/1, Switch1/3
  IM/1 -> Relational Operator/2, Switch1/1, Switch/3
  Relational Operator/1 -> Switch/2, Switch1/2, Switch2/2, Switch3/2
  Switch/1 -> OA/1
  Switch1/1 -> OB/1
  SP/1 -> Switch3/3, Switch2/1
  SM/1 -> Switch3/1, Switch2/3
  Switch2/1 -> QA/1
  Switch3/1 -> QB/1

== system AVIC_model/2値3次 NSDEM/NSDEM_3rd/Sort16/XSW8 ==
  IP : Inport
  IM : Inport  Port=2
  SP : Inport  Port=3
  SM : Inport  Port=4
  Relational Operator : RelationalOperator  Operator=<  OutDataTypeStr=boolean
  Switch{,1..3} (4 alike) : Switch  Criteria=u2 > Threshold
  OA : Outport
  OB : Outport  Port=2
  QA : Outport  Port=3
  QB : Outport  Port=4
  wires:
  Switch3/1 -> QB/1
  Switch2/1 -> QA/1
  SM/1 -> Switch2/3, Switch3/1
  SP/1 -> Switch2/1, Switch3/3
  Switch1/1 -> OB/1
  Switch/1 -> OA/1
  Relational Operator/1 -> Switch3/2, Switch2/2, Switch1/2, Switch/2
  IM/1 -> Switch/3, Switch1/1, Relational Operator/2
  IP/1 -> Switch1/3, Switch/1, Relational Operator/1

== system AVIC_model/2値3次 NSDEM/NSDEM_3rd/Sort16/XSW80 ==
  IM : Inport
  IP : Inport  Port=2
  SM : Inport  Port=3
  SP : Inport  Port=4
  Relational Operator : RelationalOperator  Operator=<  OutDataTypeStr=boolean
  Switch{,1..3} (4 alike) : Switch  Criteria=u2 > Threshold
  OB : Outport
  OA : Outport  Port=2
  QB : Outport  Port=3
  QA : Outport  Port=4
  wires:
  Switch3/1 -> QB/1
  Switch2/1 -> QA/1
  SM/1 -> Switch2/3, Switch3/1
  SP/1 -> Switch2/1, Switch3/3
  Switch1/1 -> OB/1
  Switch/1 -> OA/1
  Relational Operator/1 -> Switch3/2, Switch2/2, Switch1/2, Switch/2
  IM/1 -> Switch/3, Switch1/1, Relational Operator/2
  IP/1 -> Switch1/3, Switch/1, Relational Operator/1

== system AVIC_model/2値3次 NSDEM/NSDEM_3rd/Sort16/XSW81 ==
  IM : Inport
  IP : Inport  Port=2
  SM : Inport  Port=3
  SP : Inport  Port=4
  Relational Operator : RelationalOperator  Operator=<  OutDataTypeStr=boolean
  Switch{,1..3} (4 alike) : Switch  Criteria=u2 > Threshold
  OB : Outport
  OA : Outport  Port=2
  QB : Outport  Port=3
  QA : Outport  Port=4
  wires:
  Switch3/1 -> QB/1
  Switch2/1 -> QA/1
  SM/1 -> Switch2/3, Switch3/1
  SP/1 -> Switch2/1, Switch3/3
  Switch1/1 -> OB/1
  Switch/1 -> OA/1
  Relational Operator/1 -> Switch3/2, Switch2/2, Switch1/2, Switch/2
  IM/1 -> Switch/3, Switch1/1, Relational Operator/2
  IP/1 -> Switch1/3, Switch/1, Relational Operator/1

== system AVIC_model/2値3次 NSDEM/NSDEM_3rd/Sort16/XSW9 ==
  IP : Inport
  IM : Inport  Port=2
  SP : Inport  Port=3
  SM : Inport  Port=4
  Relational Operator : RelationalOperator  Operator=<  OutDataTypeStr=boolean
  Switch{,1..3} (4 alike) : Switch  Criteria=u2 > Threshold
  OA : Outport
  OB : Outport  Port=2
  QA : Outport  Port=3
  QB : Outport  Port=4
  wires:
  IP/1 -> Relational Operator/1, Switch/1, Switch1/3
  IM/1 -> Relational Operator/2, Switch1/1, Switch/3
  Relational Operator/1 -> Switch/2, Switch1/2, Switch2/2, Switch3/2
  Switch/1 -> OA/1
  Switch1/1 -> OB/1
  SP/1 -> Switch3/3, Switch2/1
  SM/1 -> Switch3/1, Switch2/3
  Switch2/1 -> QA/1
  Switch3/1 -> QB/1
